simulink library "driver_interface_lib"  (R2022b)
settings: Solver=VariableStepAuto  StartTime=0.0  StopTime=10.0  RelTol=1e-3
libraries: $bdroot x3, simulink x1
settings Model: Creator=dr_pa  LastModifiedBy=dr_pa

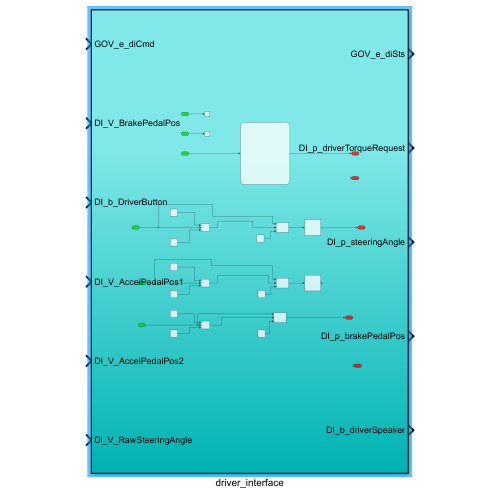
[thumbnail: Simulink's stored preview of the top-level diagram]
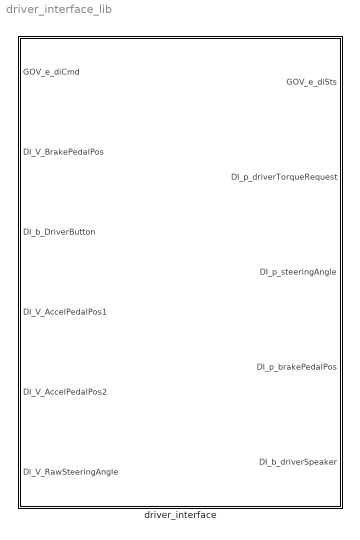
== system driver_interface_lib ==
  driver_interface : Subsystem

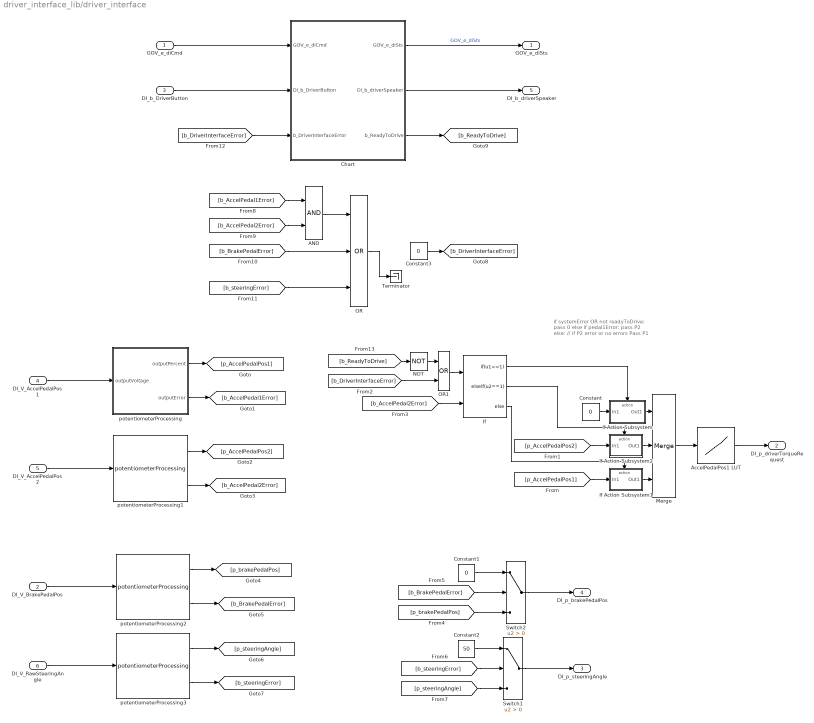
== system driver_interface_lib/driver_interface ==
  note: if systemError OR not readyToDrive:
      | 	pass 0
      | else if pedal1Error:
      | 	pass P2
      | else: // if P2 error or no errors
      | 	Pass P1
  GOV_e_diCmd : Inport
  DI_V_BrakePedalPos : Inport  Port=2
  DI_b_DriverButton : Inport  Port=3
  DI_V_AccelPedalPos1 : Inport  Port=4
  DI_V_AccelPedalPos2 : Inport  Port=5
  Dl_V_RawSteeringAngle : Inport  Port=6
  AND : Logic  AllPortsSameDT=off  OutDataTypeStr=boolean
  AccelPedalPos1 LUT : Lookup_n-D  NumberOfTableDimensions=1  BreakpointsForDimension1=[0 5 10 15 20 25 30 35 40 45 50 55 60 65 70 75 80 85 90 95 100]  Table=[0 5 10 15 20 25 30 35 40 45 50 55 60 65 70 75 80 85 90 95 100]  InternalRulePriority=Speed  RndMeth=Simplest
  Chart : Stateflow chart  TreatAsAtomicUnit=on
  Constant : Constant  Value=0  OutDataTypeStr=single
  Constant1 : Constant  Value=0  OutDataTypeStr=single
  Constant2 : Constant  Value=50  OutDataTypeStr=single
  Constant3 : Constant  Value=0  OutDataTypeStr=boolean
  If : If  NumInputs=2  IfExpression=u1==1  ElseIfExpressions=u2==1
  If Action Subsystem : Subsystem  TreatAsAtomicUnit=on
  If Action Subsystem1 : Subsystem  TreatAsAtomicUnit=on
  If Action Subsystem2 : Subsystem  TreatAsAtomicUnit=on
  Merge : Merge  Inputs=3
  NOT : Logic  Operator=NOT  IconShape=distinctive  AllPortsSameDT=off  OutDataTypeStr=boolean
  OR : Logic  Operator=OR  Inputs=3  AllPortsSameDT=off  OutDataTypeStr=boolean
  OR1 : Logic  Operator=OR  AllPortsSameDT=off  OutDataTypeStr=boolean
  Switch1 : Switch  Criteria=u2 > Threshold  SaturateOnIntegerOverflow=off  InputSameDT=off
  Switch2 : Switch  Criteria=u2 > Threshold  SaturateOnIntegerOverflow=off  InputSameDT=off
  Terminator : Terminator
  potentiometerProcessing : Subsystem
  potentiometerProcessing1 : $bdroot/driver_interface/potentiometerProcessing  SystemSampleTime=-1  VariantActivationTime=update diagram  Latency=0  AutoFrameSizeCalculation=off
  potentiometerProcessing2 : $bdroot/driver_interface/potentiometerProcessing  SystemSampleTime=-1  VariantActivationTime=update diagram  Latency=0  AutoFrameSizeCalculation=off
  potentiometerProcessing3 : $bdroot/driver_interface/potentiometerProcessing  SystemSampleTime=-1  VariantActivationTime=update diagram  Latency=0  AutoFrameSizeCalculation=off
  GOV_e_diSts : Outport
  DI_p_driverTorqueRequest : Outport  Port=2
  DI_p_steeringAngle : Outport  Port=3
  DI_p_brakePedalPos : Outport  Port=4
  DI_b_driverSpeaker : Outport  Port=5
  wires:
  Chart/1(GOV_e_diSts) -> GOV_e_diSts/1  "GOV_e_diSts"
  AccelPedalPos1 LUT/1 -> DI_p_driverTorqueRequest/1
  DI_V_AccelPedalPos1/1 -> potentiometerProcessing/1(outputVoltage)
  DI_b_DriverButton/1 -> Chart/2(DI_b_DriverButton)
  GOV_e_diCmd/1 -> Chart/1(GOV_e_diCmd)
  DI_V_AccelPedalPos2/1 -> potentiometerProcessing1/1
  Merge/1 -> AccelPedalPos1 LUT/1
  potentiometerProcessing/1(outputPercent) -> [p_AccelPedalPos1]
  potentiometerProcessing/2(outputError) -> [b_AccelPedal1Error]
  potentiometerProcessing1/1 -> [p_AccelPedalPos2]
  potentiometerProcessing1/2 -> [b_AccelPedal2Error]
  potentiometerProcessing2/2 -> [b_BrakePedalError]
  potentiometerProcessing2/1 -> [p_brakePedalPos]
  DI_V_BrakePedalPos/1 -> potentiometerProcessing2/1
  Dl_V_RawSteeringAngle/1 -> potentiometerProcessing3/1
  potentiometerProcessing3/1 -> [p_steeringAngle]
  potentiometerProcessing3/2 -> [b_steeringError]
  If Action Subsystem/1(Out1) -> Merge/1
  If/1 -> If Action Subsystem/Action
  If Action Subsystem2/1(Out1) -> Merge/2
  If Action Subsystem1/1(Out1) -> Merge/3
  [p_AccelPedalPos1] -> If Action Subsystem1/1(In1)
  [p_AccelPedalPos2] -> If Action Subsystem2/1(In1)
  [b_AccelPedal2Error] -> If/2
  [b_BrakePedalError] -> Switch2/2
  Constant1/1 -> Switch2/1
  [p_brakePedalPos] -> Switch2/3
  Switch2/1 -> DI_p_brakePedalPos/1
  Constant2/1 -> Switch1/1
  Switch1/1 -> DI_p_steeringAngle/1
  [b_steeringError] -> Switch1/2
  [p_steeringAngle] -> Switch1/3
  [b_AccelPedal2Error] -> AND/2
  [b_AccelPedal1Error] -> AND/1
  AND/1 -> OR/1
  [b_BrakePedalError] -> OR/2
  [b_steeringError] -> OR/3
  OR/1 -> Terminator/1
  [b_DriverInterfaceError] -> Chart/3(b_DriverInterfaceError)
  Chart/2(DI_b_driverSpeaker) -> DI_b_driverSpeaker/1
  Constant/1 -> If Action Subsystem/1(In1)
  If/2 -> If Action Subsystem2/Action
  If/3 -> If Action Subsystem1/Action
  Chart/3(b_ReadyToDrive) -> [b_ReadyToDrive]
  OR1/1 -> If/1
  [b_DriverInterfaceError] -> OR1/2
  [b_ReadyToDrive] -> NOT/1
  NOT/1 -> OR1/1
  Constant3/1 -> [b_DriverInterfaceError]

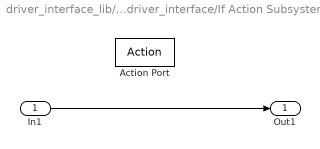
== system driver_interface_lib/driver_interface/If Action Subsystem ==
  In1 : Inport
  Action Port : ActionPort  ActionPortLabel=if(u1==1)
  Out1 : Outport
  wires:
  In1/1 -> Out1/1

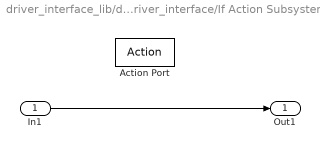
== system driver_interface_lib/driver_interface/If Action Subsystem1 ==
  In1 : Inport
  Action Port : ActionPort  ActionPortLabel=else
  Out1 : Outport
  wires:
  In1/1 -> Out1/1

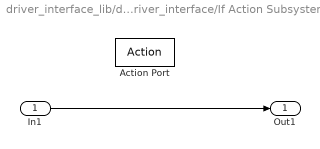
== system driver_interface_lib/driver_interface/If Action Subsystem2 ==
  In1 : Inport
  Action Port : ActionPort  ActionPortLabel=elseif(u2==1)
  Out1 : Outport
  wires:
  In1/1 -> Out1/1

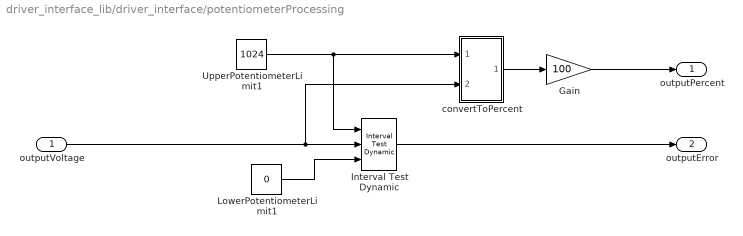
== system driver_interface_lib/driver_interface/potentiometerProcessing ==
  outputVoltage : Inport
  Gain : Gain  Gain=100
  Interval Test Dynamic : simulink/Logic and Bit Operations/Interval Test Dynamic  IntervalClosedRight=on  IntervalClosedLeft=on  OutDataTypeStr=boolean
  LowerPotentiometerLimit1 : Constant  Value=0  OutDataTypeStr=single
  UpperPotentiometerLimit1 : Constant  Value=1024  OutDataTypeStr=single
  convertToPercent : Subsystem
  outputPercent : Outport
  outputError : Outport  Port=2
  wires:
  LowerPotentiometerLimit1/1 -> Interval Test Dynamic/3
  UpperPotentiometerLimit1/1 -> Interval Test Dynamic/1, convertToPercent/1(In1)
  outputVoltage/1 -> Interval Test Dynamic/2, convertToPercent/2(In2)
  Interval Test Dynamic/1 -> outputError/1
  convertToPercent/1(Out1) -> Gain/1
  Gain/1 -> outputPercent/1

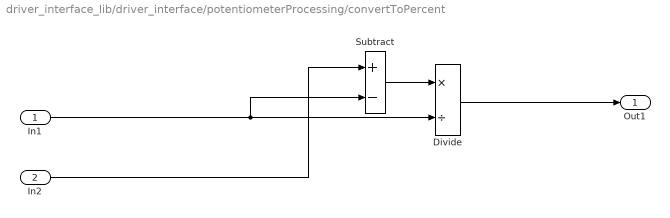
== system driver_interface_lib/driver_interface/potentiometerProcessing/convertToPercent ==
  In1 : Inport
  In2 : Inport  Port=2
  Divide : Product  Inputs=*/
  Subtract : Sum  Inputs=+-
  Out1 : Outport
  wires:
  Divide/1 -> Out1/1
  Subtract/1 -> Divide/1
  In2/1 -> Subtract/1
  In1/1 -> Divide/2, Subtract/2

== stateflow chart driver_interface_lib/driver_interface/Chart ==
  state INIT
    en:
    GOV_e_diSts = DI_STATUSES.DI_STS_INIT;
    b_ReadyToDrive=false;
    DI_b_driverSpeaker = false;
  state DI_running
    state Waiting_for_driver
      en:
      GOV_e_diSts = ...
      DI_STATUSES.WAITING_FOR_DRVR;
    state Driver_requested_start
      en:
      GOV_e_diSts = DI_STATUSES.DRV_START_REQ;
    state Ready_to_drive
      en:
      b_ReadyToDrive = true;
      GOV_e_diSts = DI_RUNNING;
      state SpeakerOn_
        en:
        DI_b_driverSpeaker = true;
      state SpeakerOff
        en:
        DI_b_driverSpeaker = false;
      (default) -> SpeakerOn_
      SpeakerOn_ -> SpeakerOff : after(2,sec)
    Waiting_for_driver -> Driver_requested_start : [DI_b_DriverButton==1]
    Driver_requested_start -> Ready_to_drive : [GOV_e_diCmd ==...
        |  DI_CMD.READY_TO_DRIVE]
  state DI_error
    en:
    GOV_e_diSts = DI_STATUSES.DI_ERROR;
  state Vehicle_coasting
    en:
    b_ReadyToDrive = false;
    GOV_e_diSts = DI_STATUSES.DI_IDLE;
  (default) -> INIT
  INIT -> Waiting_for_driver
  DI_running -> DI_error : [b_DriverInterfaceError==1]
  Ready_to_drive -> Vehicle_coasting : [GOV_e_diCmd ==...
      |  DI_CMD.SYSTEM_ERROR]
  data: GOV_e_diCmd input Enum: DI_CMD; DI_b_DriverButton input; GOV_e_diSts output Enum: DI_STATUSES size=1; b_DriverInterfaceError input; DI_b_driverSpeaker output boolean; b_ReadyToDrive output boolean
